simulink model "Part_3_Large_signal_model_with_controller"  (R2023b)
settings: Solver=ode4  StartTime=0.0  StopTime=10.0  FixedStep=0.0001  RelTol=1e-3
values from neighbouring files (symbols this model uses):
  J = 0.02    [Part_1_Solving_for_operating_points.m]
  Lr = 0.005974 + M    (= 0.311524)    [Part_1_Solving_for_operating_points.m]
  M = 0.30555    [Part_1_Solving_for_operating_points.m]
  np = 2    [Part_1_Solving_for_operating_points.m]
  Rr = 1 + 038 * 10^-3    (= 1.038)    [Part_1_Solving_for_operating_points.m]
  Rs = 1 + 300 * 10^-3    (= 1.3)    [Part_1_Solving_for_operating_points.m]
  sigma = (Ls *Lr - M^2)/(Lr)    (= 0.0118334384381)    [Part_1_Solving_for_operating_points.m]
libraries: slpidlib x2
settings Model: Creator=Santhosh  LastModifiedBy=Santhosh

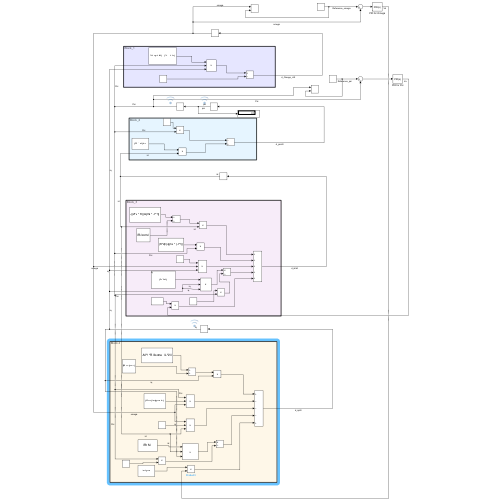
[thumbnail: Simulink's stored preview of the top-level diagram]
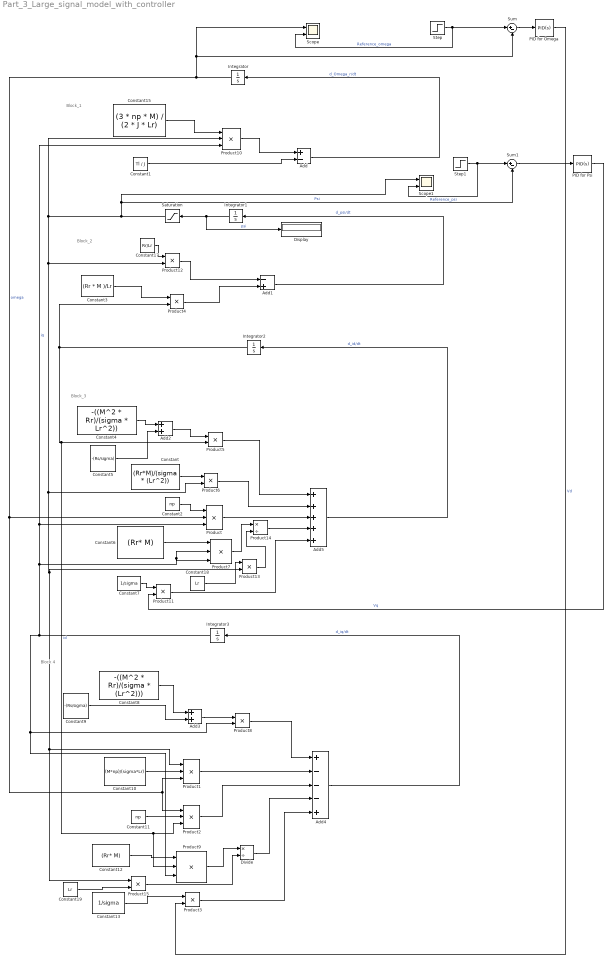
== system Part_3_Large_signal_model_with_controller ==
  note: Block_3
  note: Block_1
  note: Block 4
  note: Block_2
  Add : Sum  Inputs=+-
  Add1 : Sum  Inputs=-+
  Add2 : Sum
  Add3 : Sum
  Add4 : Sum  Inputs=+---+
  Add5 : Sum  Inputs=5
  Constant : Constant  Value=(Rr*M)/(sigma * (Lr^2))
  Constant1 : Constant  Value=Tl / J
  Constant10 : Constant  Value=(M*np)/(sigma*Lr)
  Constant11 : Constant  Value=np
  Constant12 : Constant  Value=(Rr* M)
  Constant13 : Constant  Value=1/sigma
  Constant15 : Constant  Value=(3 * np * M) / (2 * J * Lr)
  Constant17 : Constant  Value=Rr/Lr
  Constant18 : Constant  Value=Lr
  Constant19 : Constant  Value=Lr
  Constant2 : Constant  Value=np
  Constant3 : Constant  Value=(Rr * M )/Lr
  Constant4 : Constant  Value=-((M^2 * Rr)/(sigma * Lr^2))
  Constant5 : Constant  Value=-(Rs/sigma)
  Constant6 : Constant  Value=(Rr* M)
  Constant7 : Constant  Value=1/sigma
  Constant8 : Constant  Value=-((M^2 * Rr)/(sigma * (Lr^2)))
  Constant9 : Constant  Value=-(Rs/sigma)
  Display : Display
  Divide : Product  Inputs=*/
  Integrator{,1..3} (4 alike) : Integrator
  PID for Omega : slpidlib/PID Controller  Controller=PID  Form=Parallel  TimeDomain=Continuous-time  UseExternalTs=off  SampleTime=-1  IntegratorMethod=Forward Euler  FilterMethod=Forward Euler  ControllerParametersSource=internal  P=4  I=10.255  UseKiTs=off  D=0  N=100  UseFilter=on  TunerSelectOption=Transfer Function Based (PID Tuner App)  InitialConditionSource=internal  InitialConditionForIntegrator=0  InitialConditionForFilter=0  DifferentiatorICPrevScaledInput=0  ExternalReset=none  TrackingMode=off  Kt=1  LimitOutput=off  SatLimitsSource=internal  UpperSaturationLimit=inf  LowerSaturationLimit=-inf  LinearizeAsGain=on  AntiWindupMode=none  Kb=1  LimitIntegrator=off  UpperIntegratorSaturationLimit=inf  LowerIntegratorSaturationLimit=-inf  POutMin=[]  POutMax=[]  IOutMin=[]  IOutMax=[]  DOutMin=[]  DOutMax=[]  NOutMin=[]  NOutMax=[]  SumOutMin=[]  SumOutMax=[]  SaturationOutMin=[]  SaturationOutMax=[]  PParamMin=[]  PParamMax=[]  IParamMin=[]  IParamMax=[]  DParamMin=[]  DParamMax=[]  NParamMin=[]  NParamMax=[]  KbParamMin=[]  KbParamMax=[]  KtParamMin=[]  KtParamMax=[]  KbOutMin=[]  KbOutMax=[]  KtOutMin=[]  KtOutMax=[]  IntegratorOutMin=[]  IntegratorOutMax=[]  FilterOutMin=[]  FilterOutMax=[]  SumI1OutMin=[]  SumI1OutMax=[]  SumI2OutMin=[]  SumI2OutMax=[]  SumI3OutMin=[]  SumI3OutMax=[]  SumI4OutMin=[]  SumI4OutMax=[]  SumDOutMin=[]  SumDOutMax=[]  DifferentiatorOutMin=[]  DifferentiatorOutMax=[]  FilterDiffOutCoefMin=[]  FilterDiffOutCoefMax=[]  ReciprocalOutMin=[]  ReciprocalOutMax=[]  SumDenOutMin=[]  SumDenOutMax=[]  SumNumOutMin=[]  SumNumOutMax=[]  DivideOutMin=[]  DivideOutMax=[]  UdiffTsProdOutMin=[]  UdiffTsProdOutMax=[]  NTsProdOutMin=[]  NTsProdOutMax=[]  UintegralTsProdOutMin=[]  UintegralTsProdOutMax=[]  UngainTsProdOutMin=[]  UngainTsProdOutMax=[]  ClampingZeroOutDataTypeStr=Inherit: Inherit via back propagation  ClampingZeroOutMin=[]  ClampingZeroOutMax=[]  FilterDenConstantOutDataTypeStr=Inherit: Inherit via back propagation  FilterDenConstantOutMin=[]  FilterDenConstantOutMax=[]  PCopyOutDataTypeStr=Inherit: Inherit via back propagation  PCopyOutMin=[]  PCopyOutMax=[]  NCopyOutDataTypeStr=Inherit: Inherit via back propagation  NCopyOutMin=[]  NCopyOutMax=[]  IntegratorContinuousStateAttributes=''  IntegratorStateMustResolveToSignalObject=off  IntegratorRTWStateStorageClass=Auto  FilterContinuousStateAttributes=''  FilterStateMustResolveToSignalObject=off  FilterRTWStateStorageClass=Auto  ParallelPVariant=InternalParameters  IdealPVariant=Disabled  IVariant=InternalParameters  DVariant=InternalParameters  IntegratorVariant=Continuous  SatVariant=Disabled  AWVariant=Passthrough  PCopyVariant=Disabled  TRVariant=Disabled  FdbkBlocksVariant=Forward  IdealPFdbkVariant=Disabled  SatFdbkVariant=Disabled  DerivativeFilterVariant=ContFilter  NVariant=InternalParameters  NCopyVariant=Disabled  FilterICVariant=InternalICsFilter  IntegratorICVariant=InternalICs  ExternalResetVariant=Disabled  TRSumVariant=Passthrough  SumFdbkVariant=Disabled  SumVariant=Sum_PID  TsampFilterVariant=InternalTs  TsampNgainVariant=Passthrough  TsampIntegralVariant=Disabled_SignalSpec  ExternalSaturationOutDataTypeStr=Inherit: Same as second input
  PID for Psi : slpidlib/PID Controller  Controller=PID  Form=Parallel  TimeDomain=Continuous-time  UseExternalTs=off  SampleTime=-1  IntegratorMethod=Forward Euler  FilterMethod=Forward Euler  ControllerParametersSource=internal  P=271  I=981  UseKiTs=off  D=0  N=100  UseFilter=on  TunerSelectOption=Transfer Function Based (PID Tuner App)  InitialConditionSource=internal  InitialConditionForIntegrator=0  InitialConditionForFilter=0  DifferentiatorICPrevScaledInput=0  ExternalReset=none  TrackingMode=off  Kt=1  LimitOutput=off  SatLimitsSource=internal  UpperSaturationLimit=inf  LowerSaturationLimit=-inf  LinearizeAsGain=on  AntiWindupMode=none  Kb=1  LimitIntegrator=off  UpperIntegratorSaturationLimit=inf  LowerIntegratorSaturationLimit=-inf  POutMin=[]  POutMax=[]  IOutMin=[]  IOutMax=[]  DOutMin=[]  DOutMax=[]  NOutMin=[]  NOutMax=[]  SumOutMin=[]  SumOutMax=[]  SaturationOutMin=[]  SaturationOutMax=[]  PParamMin=[]  PParamMax=[]  IParamMin=[]  IParamMax=[]  DParamMin=[]  DParamMax=[]  NParamMin=[]  NParamMax=[]  KbParamMin=[]  KbParamMax=[]  KtParamMin=[]  KtParamMax=[]  KbOutMin=[]  KbOutMax=[]  KtOutMin=[]  KtOutMax=[]  IntegratorOutMin=[]  IntegratorOutMax=[]  FilterOutMin=[]  FilterOutMax=[]  SumI1OutMin=[]  SumI1OutMax=[]  SumI2OutMin=[]  SumI2OutMax=[]  SumI3OutMin=[]  SumI3OutMax=[]  SumI4OutMin=[]  SumI4OutMax=[]  SumDOutMin=[]  SumDOutMax=[]  DifferentiatorOutMin=[]  DifferentiatorOutMax=[]  FilterDiffOutCoefMin=[]  FilterDiffOutCoefMax=[]  ReciprocalOutMin=[]  ReciprocalOutMax=[]  SumDenOutMin=[]  SumDenOutMax=[]  SumNumOutMin=[]  SumNumOutMax=[]  DivideOutMin=[]  DivideOutMax=[]  UdiffTsProdOutMin=[]  UdiffTsProdOutMax=[]  NTsProdOutMin=[]  NTsProdOutMax=[]  UintegralTsProdOutMin=[]  UintegralTsProdOutMax=[]  UngainTsProdOutMin=[]  UngainTsProdOutMax=[]  ClampingZeroOutDataTypeStr=Inherit: Inherit via back propagation  ClampingZeroOutMin=[]  ClampingZeroOutMax=[]  FilterDenConstantOutDataTypeStr=Inherit: Inherit via back propagation  FilterDenConstantOutMin=[]  FilterDenConstantOutMax=[]  PCopyOutDataTypeStr=Inherit: Inherit via back propagation  PCopyOutMin=[]  PCopyOutMax=[]  NCopyOutDataTypeStr=Inherit: Inherit via back propagation  NCopyOutMin=[]  NCopyOutMax=[]  IntegratorContinuousStateAttributes=''  IntegratorStateMustResolveToSignalObject=off  IntegratorRTWStateStorageClass=Auto  FilterContinuousStateAttributes=''  FilterStateMustResolveToSignalObject=off  FilterRTWStateStorageClass=Auto  ParallelPVariant=InternalParameters  IdealPVariant=Disabled  IVariant=InternalParameters  DVariant=InternalParameters  IntegratorVariant=Continuous  SatVariant=Disabled  AWVariant=Passthrough  PCopyVariant=Disabled  TRVariant=Disabled  FdbkBlocksVariant=Forward  IdealPFdbkVariant=Disabled  SatFdbkVariant=Disabled  DerivativeFilterVariant=ContFilter  NVariant=InternalParameters  NCopyVariant=Disabled  FilterICVariant=InternalICsFilter  IntegratorICVariant=InternalICs  ExternalResetVariant=Disabled  TRSumVariant=Passthrough  SumFdbkVariant=Disabled  SumVariant=Sum_PID  TsampFilterVariant=InternalTs  TsampNgainVariant=Passthrough  TsampIntegralVariant=Disabled_SignalSpec  ExternalSaturationOutDataTypeStr=Inherit: Same as second input
  Product{,1..2,10} (4 alike) : Product  Inputs=3
  Product{3..6,8,11..13,15} (9 alike) : Product
  Product14 : Product  Inputs=*/
  Product7 : Product  Inputs=***
  Product9 : Product  Inputs=***
  Saturation : Saturate  UpperLimit=1  LowerLimit=0.00001
  Scope : Scope  NumInputPorts=2
  Scope1 : Scope  NumInputPorts=2
  Step : Step  After=180  SampleTime=0
  Step1 : Step  After=0.5  SampleTime=0
  Sum : Sum  Inputs=|+-
  Sum1 : Sum  Inputs=|+-
  wires:
  Add2/1 -> Product5/1
  Integrator2/1 -> Product9/2, Product2/3, Product5/2, Product4/2  "id"
  Integrator3/1 -> Product9/3, Product8/2, Product7/2, Product7/3, Product/3, Product10/3  "iq"
  Product13/1 -> Product14/2
  Divide/1 -> Add4/4
  Constant18/1 -> Product13/1
  Product5/1 -> Add5/1
  Add/1 -> Integrator/1  "d_Omega_r/dt"
  Constant1/1 -> Add/2
  Product12/1 -> Add1/1
  Product4/1 -> Add1/2
  Constant5/1 -> Add2/2
  Constant15/1 -> Product10/1
  Constant4/1 -> Add2/1
  Product/1 -> Add5/3
  Constant3/1 -> Product4/1
  Constant/1 -> Product6/1
  Product11/1 -> Add5/5
  Product6/1 -> Add5/2
  Add1/1 -> Integrator1/1  "d_psi/dt"
  Product2/1 -> Add4/3
  Constant6/1 -> Product7/1
  Add4/1 -> Integrator3/1  "d_iq/dt"
  Constant8/1 -> Add3/1
  Constant13/1 -> Product3/1
  Product9/1 -> Divide/1
  Add5/1 -> Integrator2/1  "d_id/dt"
  Product10/1 -> Add/1
  Product15/1 -> Divide/2
  Constant12/1 -> Product9/1
  Add3/1 -> Product8/1
  Product8/1 -> Add4/1
  Product1/1 -> Add4/2
  Product7/1 -> Product14/1
  Constant11/1 -> Product2/2
  Constant7/1 -> Product11/1
  Integrator/1 -> Product2/1, Product1/3, Product/2, Sum/2, Scope/1  "omega"
  Product14/1 -> Add5/4
  Constant17/1 -> Product12/1
  Product3/1 -> Add4/5
  Constant10/1 -> Product1/2
  Constant2/1 -> Product/1
  Constant19/1 -> Product15/2
  Constant9/1 -> Add3/2
  Step/1 -> Scope/2, Sum/1  "Reference_omega"
  Sum/1 -> PID for Omega/1
  Step1/1 -> Scope1/2, Sum1/1  "Reference_psi"
  Sum1/1 -> PID for Psi/1
  Integrator1/1 -> Display/1, Saturation/1  "psi"
  Saturation/1 -> Sum1/2, Scope1/1, Product10/2, Product12/2, Product15/1, Product1/1, Product13/2, Product6/2  "Psi"
  PID for Omega/1 -> Product3/2  "Vd"
  PID for Psi/1 -> Product11/2  "Vq"
